simulink model "vehicle_model_controller_ref"  (R2020b)
settings: Solver=VariableStepAuto  StartTime=0.0  StopTime=180  FixedStep=0.001  RelTol=1e-3
model workspace (MAT data in the model file):
  understeer_gradient = 0.05
undefined symbols (not defined in the file or in its folder): front_forces, rear_forces
libraries: fl_lib x24, nesl_utility x20, sdl_lib x8, autolibmappedmotor x4, vehdynlibsteering x1, pid_lib x1, autolibshared x1, autolibdatasheetbattery x1
(part 1 of 4)
settings Model: TunableVars=F_sv,F_x_ij,F_x_ij_max,F_y_fl,F_y_fr,F_y_ij,F_y_rl,F_y_rr,J_z,K_1,K_2,LB,PID,R,T_x_ij,UP,delta,driver_input,err,l,l_f,l_r,linsol,s,s_f,s_r,x,x_1,x_2,x_3,x_4,y,y_1,y_2,y_3,y_4  TunableVarsStorageClass=Auto,Auto,Auto,Auto,Auto,Auto,Auto,Auto,Auto,Auto,Auto,Auto,Auto,Auto,Auto,Auto,Auto,Auto,Auto,Auto,Auto,Auto,Auto,Auto,Auto,Auto,Auto,Auto,Auto,Auto,Auto,Auto,Auto,Auto,Auto,Auto  TunableVarsTypeQualifier=,,,,,,,,,,,,,,,,,,,,,,,,,,,,,,,,,,,  ParameterArgumentNames=understeer_gradient  OrderedModelArguments=off  Creator=True  LastModifiedBy=Inver
settings DataIOCC: ExternalInput=Sheet1.getElement('driver_input'),Sheet1.getElement('batt_temp'),Sheet1.getElement('steering_angle'),Sheet1.getElement('wind z'),Sheet1.getElement('b_FL'),Sheet1.getElement('wind x'),Sheet1.getElement('wind y'),Sheet1.getElement('b_FR'),Sheet1.getElement('b_RL'),Sheet1.getElement('b_RR')  LoadExternalInput=on
settings OptimizationCC: DefaultParameterBehavior=Inlined  GainParamInheritBuiltInType=on  UseFloatMulNetSlope=on  InlineInvariantSignals=on  OptimizeBlockIOStorage=off  BufferReuse=off  EnhancedBackFolding=on  PassReuseOutputArgsThreshold=0  EfficientFloat2IntCast=on  EfficientMapNaN2IntZero=off  OptimizeBlockOrder=speed  DifferentSizesBufferReuse=on
settings DebuggingCC: SolverPrmCheckMsg=error  ParameterTunabilityLossMsg=error  ArithmeticOperatorsInVariantConditions=warning
settings HardwareCC: TargetBitPerPointer=64  TargetBitPerSizeT=64  TargetBitPerPtrDiffT=64  TargetLongLongMode=on  TargetIntDivRoundTo=Zero  TargetEndianess=LittleEndian  TargetWordSize=64  TargetHWDeviceType=MATLAB Host  ProdEqTarget=off
settings SFSimCC: SimUserIncludeDirs=$matlabroot$\toolbox\rtw\rtwdemos\EmbeddedCoderOverview\  SimAnalyzeCustomCode=on  MATLABDynamicMemAlloc=off  CustomCodeUndefinedFunction=UseInterfaceOnly  SimTargetLang=C++
settings RTWCC: Description=Rapid Simulation Target  SystemTargetFile=rsim.tlc  GenCodeOnly=on  TemplateMakefile=rsim_default_tmf  GenerateReport=on  BuildConfiguration=Faster Runs  LaunchReport=on  CheckMdlBeforeBuild=Warning
settings CodeAppCC: ForceParamTrailComments=on  OperatorAnnotations=on
settings RSimTargetCC: TargetLangStandard=C99 (ISO)
settings ConfigComp: CovScope=ReferencedModels
settings SimscapeCC: SimscapeLogType=local

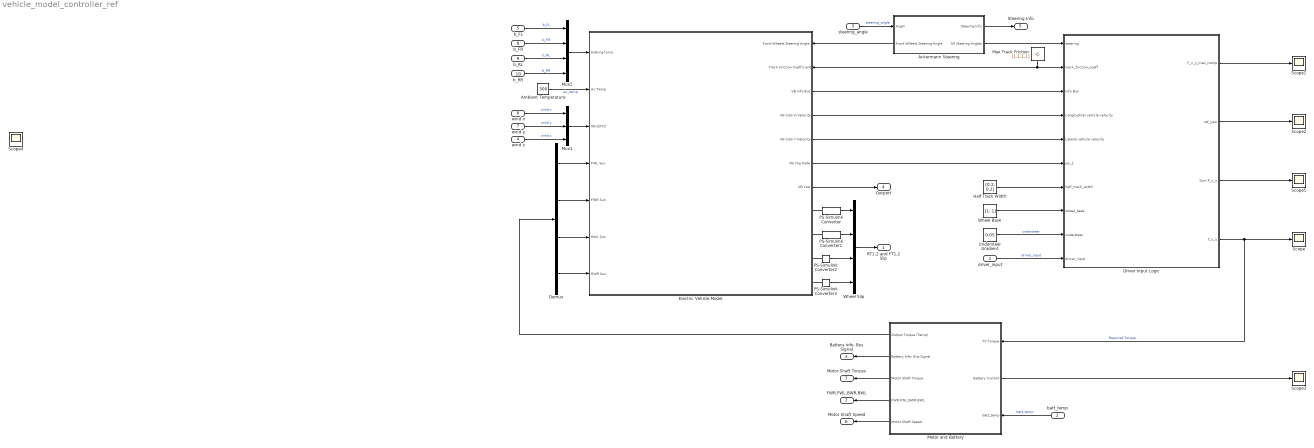
== system vehicle_model_controller_ref ==
  driver_input : Inport  Interpolate=off
  batt_temp : Inport  Port=2
  steering_angle : Inport  Port=3
  wind z : Inport  Port=4
  b_FL : Inport  Port=5
  wind x : Inport  Port=6
  wind y : Inport  Port=7
  b_FR : Inport  Port=8
  b_RL : Inport  Port=9
  b_RR : Inport  Port=10
  Ackermann Steering : Subsystem
      settings: PortSchema="{\"entries\":[{\"content\":{\"sides\":[{\"content\":{\"connectorIds\":[\"In1\",\"Out3\"]},\"type\":\"ConnectorPlacement.EquallySpacedRectSide\",\"uuid\":\"7629c306-c8a5-46d9-919e-1a99248f4fd8\"},{\"content\":{\"connectorIds\":[\"Out1\",\"Out2\"],\"side\":\"RIGHT\"},\"type\":\"ConnectorPlacement.EquallySpacedRectSide\",\"uuid\":\"a1deaca9-77cb-4ffb-842f-c827aa96d417\"},{\"content\":{\"connectorIds\":[],\"side\":\"TOP\"},\"type\":\"ConnectorPlacement.EquallySpacedRectSide\",\"uuid\":\"391c149d-58be-48e2-876e-8c407e7d25f9\"},{\"content\":{\"connectorIds\":[],\"side\":\"HIDDEN\"},\"type\":\"ConnectorPlacement.EquallySpacedRectSide\",\"uuid\":\"557ca4cc-9d5d-4724-8dd0-cdc929429066\"}]},\"type\":\"ConnectorPlacement.EquallySpacedConnector\",\"uuid\":\"b8a1e7c7-7192-4f65-ab36-8db1985dd1bc\"}],\"packageUris\":[\"http://schema.mathworks.com/mf0/Connector/R2020b\"],\"version\":\"1.0\"}"
  Ambient Temperature : Constant  Value=300
  Demux : Demux
  Driver Input Logic : Subsystem
  Electric Vehicle Model : Subsystem
      settings: PortSchema="{\"entries\":[{\"content\":{\"sides\":[{\"content\":{\"connectorIds\":[\"In1\",\"In2\",\"In3\",\"In4\",\"In5\",\"In6\",\"In7\"]},\"type\":\"ConnectorPlacement.EquallySpacedRectSide\",\"uuid\":\"d116468d-7868-487f-a964-21d40fbcc809\"},{\"content\":{\"connectorIds\":[\"In8\",\"In9\",\"Out1\",\"Out2\",\"Out3\",\"Out4\",\"Out5\",\"RConn1\",\"RConn2\",\"RConn3\",\"RConn4\"],\"side\":\"RIGHT\"},\"type\":\"ConnectorPlacement.EquallySpacedRectSide\",\"uuid\":\"69901164-3ba1-4787-94a1-b6dad3f5570f\"},{\"content\":{\"connectorIds\":[],\"side\":\"TOP\"},\"type\":\"ConnectorPlacement.EquallySpacedRectSide\",\"uuid\":\"0399aa14-7cbc-406a-a0bc-5234930aa618\"},{\"content\":{\"connectorIds\":[],\"side\":\"HIDDEN\"},\"type\":\"ConnectorPlacement.EquallySpacedRectSide\",\"uuid\":\"c7425876-ea80-44ac-a5c9-676a45313985\"}]},\"type\":\"ConnectorPlacement.EquallySpacedConnector\",\"uuid\":\"33585625-d9f5-41d4-8b4d-b29cb62e09b6\"}],\"packageUris\":[\"http://schema.mathworks.com/mf0/Connector/R2020b\"],\"version\":\"1.0\"}"
  Half Track Width : Constant  Value=[0.2, 0.2]
  Max Track Friction : Constant  Value=[1,1;1,1]
  Motor and Battery : Subsystem
      settings: PortSchema="{\"entries\":[{\"content\":{\"sides\":[{\"content\":{\"connectorIds\":[\"Out2\",\"Out3\",\"Out4\",\"Out5\",\"Out6\"]},\"type\":\"ConnectorPlacement.EquallySpacedRectSide\",\"uuid\":\"d5eb6e01-74de-485f-b814-f74cf87d6300\"},{\"content\":{\"connectorIds\":[\"In1\",\"Out1\",\"In2\"],\"side\":\"RIGHT\"},\"type\":\"ConnectorPlacement.EquallySpacedRectSide\",\"uuid\":\"4e9b95b3-1238-4789-a4cc-20b236b4d536\"},{\"content\":{\"connectorIds\":[],\"side\":\"TOP\"},\"type\":\"ConnectorPlacement.EquallySpacedRectSide\",\"uuid\":\"97fc91bc-a36c-43db-88cf-61ba0348fc60\"},{\"content\":{\"connectorIds\":[],\"side\":\"HIDDEN\"},\"type\":\"ConnectorPlacement.EquallySpacedRectSide\",\"uuid\":\"c955884f-22bb-4f22-9982-ff8bef63f64d\"}]},\"type\":\"ConnectorPlacement.EquallySpacedConnector\",\"uuid\":\"927982b2-ec40-42a1-9f55-58bc607d6a22\"}],\"packageUris\":[\"http://schema.mathworks.com/mf0/Connector/R2020b\"],\"version\":\"1.0\"}"
  Mux1 : Mux  Inputs=3
  Mux2 : Mux
  PS-Simulink Converter{,1..3} (4 alike) : nesl_utility/PS-Simulink Converter  PhysicalDomain=network_engine_domain  SubClassName=ps_output  LeftPortType=input  RightPortType=output  PseudoPeriodic=off  Frequencies=[]  Unit=inherit  AffineConversion=off
  Scope{,1..5} (6 alike) : Scope
  Understeer Gradient : Constant  Value=0.05
  Wheel Base : Constant  Value=[1, 1]
  Wheel Slip : Mux
  RT1,2 and FT1,2 Slip : Outport
  FWR,FWL,BWR,BWL : Outport  Port=2
  Battery Info- Bus Signal : Outport  Port=3
  Outport : Outport  Port=4
  Steering Info : Outport  Port=5
  Motor Shaft Speed : Outport  Port=6
  Motor Shaft Torque : Outport  Port=7
  wires:
  PS-Simulink Converter/1 -> Wheel Slip/1
  PS-Simulink Converter1/1 -> Wheel Slip/2
  PS-Simulink Converter2/1 -> Wheel Slip/3
  PS-Simulink Converter3/1 -> Wheel Slip/4
  Wheel Slip/1 -> RT1,2 and FT1,2 Slip/1
  Electric Vehicle Model/5(VB Yaw) -> Outport/1
  Ambient Temperature/1 -> Electric Vehicle Model/2(Air Temp)  "air_temp"
  Electric Vehicle Model/1(VB Info Bus) -> Driver Input Logic/3(Info Bus)
  Electric Vehicle Model/2("VB CoG X-Velocity ") -> Driver Input Logic/4(Longitudinal vehicle velocity)
  Electric Vehicle Model/3(VB CoG Y-Velocity) -> Driver Input Logic/5(Lateral vehicle velocity)
  Electric Vehicle Model/4(VB Yaw Rate) -> Driver Input Logic/6(psi_1)
  Understeer Gradient/1 -> Driver Input Logic/9(understeer)  "understeer"
  driver_input/1 -> Driver Input Logic/10(driver_input)  "driver_input"
  Driver Input Logic/4(T_x_ij) -> Scope/1, Motor and Battery/1(TV Torque)  "Required Torque"
  Half Track Width/1 -> Driver Input Logic/7(half_track_width)
  Wheel Base/1 -> Driver Input Logic/8(wheel_base)
  Driver Input Logic/1(F_x_ij_max_noslip) -> Scope1/1
  Driver Input Logic/2(ref_yaw) -> Scope2/1
  wind x/1 -> Mux1/1  "wind x"
  wind y/1 -> Mux1/2  "wind y"
  wind z/1 -> Mux1/3  "wind z"
  Mux1/1 -> Electric Vehicle Model/3(WindXYZ)
  b_FR/1 -> Mux2/2  "b_FR"
  b_FL/1 -> Mux2/1  "b_FL"
  b_RL/1 -> Mux2/3  "b_RL"
  b_RR/1 -> Mux2/4  "b_RR"
  Ackermann Steering/1(Steering Info) -> Steering Info/1
  Ackermann Steering/3(Front Wheels Steering Angle) -> Electric Vehicle Model/8(Front Wheels Steering Angle)
  Ackermann Steering/2(All Steering Angles) -> Driver Input Logic/1(steering)
  Max Track Friction/1 -> Driver Input Logic/2(track_friction_coeff), Electric Vehicle Model/9(Track Friction Coefficient)
  steering_angle/1 -> Ackermann Steering/1(AngIn)  "steering_angle"
  Driver Input Logic/3(Sum F_x_ij) -> Scope5/1
  Demux/4 -> Electric Vehicle Model/7(RWR Sun)
  Demux/3 -> Electric Vehicle Model/6(RWL Sun)
  Demux/2 -> Electric Vehicle Model/5(FWR Sun)
  Demux/1 -> Electric Vehicle Model/4(FWL Sun)
  Mux2/1 -> Electric Vehicle Model/1(braking force)
  batt_temp/1 -> Motor and Battery/2(batt_temp)  "batt_temp"
  Motor and Battery/2(Output Torque (Temp)) -> Demux/1
  Motor and Battery/1(Battery Current) -> Scope3/1
  Motor and Battery/3(Battery Info- Bus Signal) -> Battery Info- Bus Signal/1
  Motor and Battery/5(FWR,FWL,BWR,BWL) -> FWR,FWL,BWR,BWL/1
  Motor and Battery/4(Motor Shaft Torque) -> Motor Shaft Torque/1
  Motor and Battery/6(Motor Shaft Speed) -> Motor Shaft Speed/1
  connections:
  PS-Simulink Converter/LConn1 -- Electric Vehicle Model/RConn1
  PS-Simulink Converter1/LConn1 -- Electric Vehicle Model/RConn2
  PS-Simulink Converter2/LConn1 -- Electric Vehicle Model/RConn3
  PS-Simulink Converter3/LConn1 -- Electric Vehicle Model/RConn4

== system vehicle_model_controller_ref/Ackermann Steering ==
  AngIn : Inport
  Bus Creator : BusCreator  Inputs=2
  Deg to Rad : Gain  Gain=pi/180
  Kinematic Steering : vehdynlibsteering/Kinematic Steering  StrgType=Ackerman  StrgRatioType=Constant  Loc=Front  NrmlFctr=1  TrckWdth=1  WhlBase=1.524  Db=0  StrgRng=1.25*pi  StrgAngBpts="[-6.2832   -5.0265   -3.7699   -2.5133   -1.2566         0    1.2566    2.5133    3.7699    5.0265    6.2832]"  StrgRatioTbl=|  StrgRatio=1  StrgArmLngth=0.1  RckCsLngth=0.5  TieRodLngth=0.248  D=0.2  PnnRadius=0.0057  PnnRadiusTbl="[0.0055    0.0055    0.0056    0.0057    0.0058    0.0057    0.0057    0.0057    0.0056    0.0055    0.0055]"  RodLngth=0.1  ParaArmLngth=0.9  aMode=2
      | [13.5000   13.3750   13.2500   13.1250   13.0000   13.0000   13.0000   13.1250   13.2500   13.3750   13.5000
      | ]
  Mux3 : Mux  Inputs=2
  Steering Info : Outport
  All Steering Angles : Outport  Port=2
  Front Wheels Steering Angle : Outport  Port=3
  wires:
  Kinematic Steering/2 -> Mux3/1
  Kinematic Steering/3 -> Mux3/2
  Kinematic Steering/1 -> Steering Info/1
  Mux3/1 -> Bus Creator/1, Front Wheels Steering Angle/1  "ackermann angles"
  Bus Creator/1 -> All Steering Angles/1
  Deg to Rad/1 -> Kinematic Steering/1, Bus Creator/2  "steering_angle"
  AngIn/1 -> Deg to Rad/1  "steering_angle"

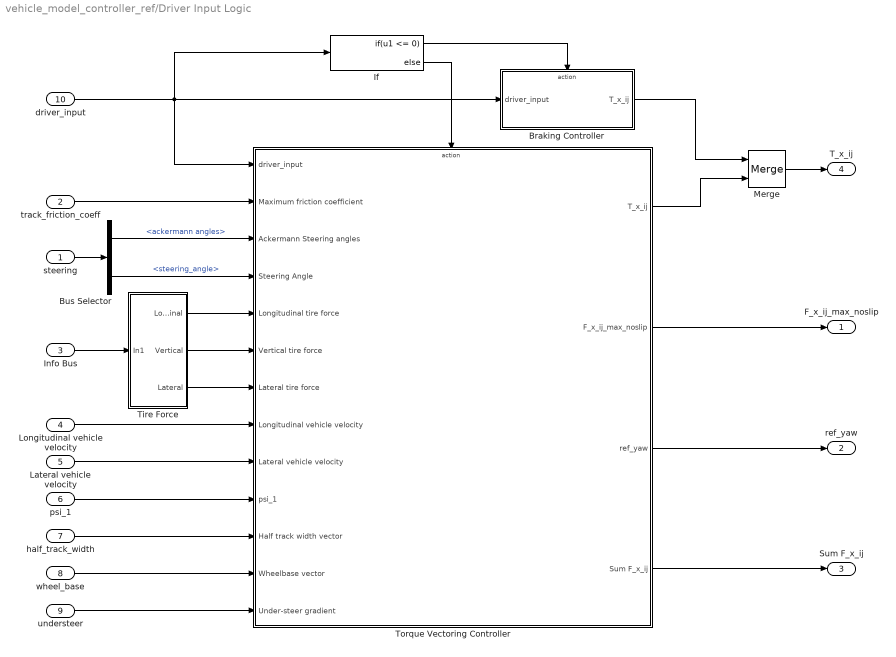
== system vehicle_model_controller_ref/Driver Input Logic ==
  steering : Inport
  track_friction_coeff : Inport  Port=2
  Info Bus : Inport  Port=3
  Longitudinal vehicle velocity : Inport  Port=4
  Lateral vehicle velocity : Inport  Port=5
  psi_1 : Inport  Port=6
  half_track_width : Inport  Port=7
  wheel_base : Inport  Port=8
  understeer : Inport  Port=9
  driver_input : Inport  Port=10
  Braking Controller : Subsystem
  Bus Selector : BusSelector  OutputSignals=ackermann angles,steering_angle
  If : If  IfExpression=u1 <= 0
  Merge : Merge
  Tire Force : Subsystem
  Torque Vectoring Controller : Subsystem
  F_x_ij_max_noslip : Outport
  ref_yaw : Outport  Port=2
  Sum F_x_ij : Outport  Port=3
  T_x_ij : Outport  Port=4
  wires:
  half_track_width/1 -> Torque Vectoring Controller/11(Half track width vector)
  understeer/1 -> Torque Vectoring Controller/13(Under-steer gradient)
  Tire Force/1(Longitudinal) -> Torque Vectoring Controller/5(Longitudinal tire force)
  Lateral vehicle velocity/1 -> Torque Vectoring Controller/9(Lateral vehicle velocity)
  wheel_base/1 -> Torque Vectoring Controller/12(Wheelbase vector)
  Longitudinal vehicle velocity/1 -> Torque Vectoring Controller/8(Longitudinal vehicle velocity)
  Tire Force/2(Vertical) -> Torque Vectoring Controller/6(Vertical tire force)
  Info Bus/1 -> Tire Force/1(In1)
  psi_1/1 -> Torque Vectoring Controller/10(psi_1)
  track_friction_coeff/1 -> Torque Vectoring Controller/2(Maximum friction coefficient)
  If/1 -> Braking Controller/Action
  Merge/1 -> T_x_ij/1
  If/2 -> Torque Vectoring Controller/Action
  Braking Controller/1(T_x_ij) -> Merge/1
  Torque Vectoring Controller/1(T_x_ij) -> Merge/2
  driver_input/1 -> Torque Vectoring Controller/1(driver_input), Braking Controller/1(driver_input), If/1
  Bus Selector/2 -> Torque Vectoring Controller/4(Steering Angle)  "<steering_angle>"
  Bus Selector/1 -> Torque Vectoring Controller/3("Ackermann Steering angles ")  "<ackermann angles>"
  Torque Vectoring Controller/2(F_x_ij_max_noslip) -> F_x_ij_max_noslip/1
  Torque Vectoring Controller/3(ref_yaw) -> ref_yaw/1
  Tire Force/3(Lateral) -> Torque Vectoring Controller/7(Lateral tire force)
  steering/1 -> Bus Selector/1
  Torque Vectoring Controller/4(Sum F_x_ij) -> Sum F_x_ij/1

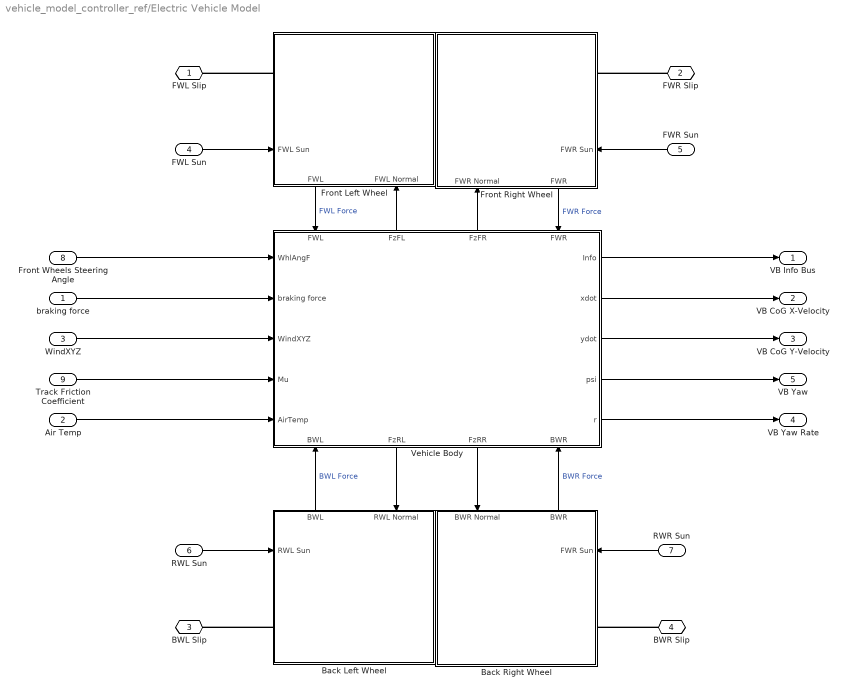
== system vehicle_model_controller_ref/Electric Vehicle Model ==
  braking force : Inport
  Air Temp : Inport  Port=2
  WindXYZ : Inport  Port=3
  FWL Sun : Inport  Port=4
  FWR Sun : Inport  Port=5
  RWL Sun : Inport  Port=6
  RWR Sun : Inport  Port=7
  Front Wheels Steering Angle : Inport  Port=8
  Track Friction Coefficient : Inport  Port=9
  Back Left Wheel : Subsystem
      settings: PortSchema="{\"entries\":[{\"content\":{\"sides\":[{\"content\":{\"connectorIds\":[\"In1\",\"LConn1\"]},\"type\":\"ConnectorPlacement.EquallySpacedRectSide\",\"uuid\":\"9f52900f-df3e-41ac-b258-782e5d4e0eaf\"},{\"content\":{\"connectorIds\":[],\"side\":\"RIGHT\"},\"type\":\"ConnectorPlacement.EquallySpacedRectSide\",\"uuid\":\"34c2d9dc-60c7-40ad-be28-599fbc039141\"},{\"content\":{\"connectorIds\":[\"Out1\",\"In2\"],\"side\":\"TOP\"},\"type\":\"ConnectorPlacement.EquallySpacedRectSide\",\"uuid\":\"1dcff801-acc8-4468-b9f1-4bf879f78c2b\"},{\"content\":{\"connectorIds\":[],\"side\":\"HIDDEN\"},\"type\":\"ConnectorPlacement.EquallySpacedRectSide\",\"uuid\":\"30765525-e7e6-43f5-8314-8ed292f1691c\"}]},\"type\":\"ConnectorPlacement.EquallySpacedConnector\",\"uuid\":\"fe63b2f8-6027-4789-9c90-5c54dbfc2a0a\"}],\"packageUris\":[\"http://schema.mathworks.com/mf0/Connector/R2020b\"],\"version\":\"1.0\"}"
  Back Right Wheel : Subsystem
      settings: PortSchema="{\"entries\":[{\"content\":{\"sides\":[{\"content\":{\"connectorIds\":[]},\"type\":\"ConnectorPlacement.EquallySpacedRectSide\",\"uuid\":\"9f52900f-df3e-41ac-b258-782e5d4e0eaf\"},{\"content\":{\"connectorIds\":[\"In2\",\"RConn1\"],\"side\":\"RIGHT\"},\"type\":\"ConnectorPlacement.EquallySpacedRectSide\",\"uuid\":\"34c2d9dc-60c7-40ad-be28-599fbc039141\"},{\"content\":{\"connectorIds\":[\"In1\",\"Out1\"],\"side\":\"TOP\"},\"type\":\"ConnectorPlacement.EquallySpacedRectSide\",\"uuid\":\"1dcff801-acc8-4468-b9f1-4bf879f78c2b\"},{\"content\":{\"connectorIds\":[],\"side\":\"HIDDEN\"},\"type\":\"ConnectorPlacement.EquallySpacedRectSide\",\"uuid\":\"30765525-e7e6-43f5-8314-8ed292f1691c\"}]},\"type\":\"ConnectorPlacement.EquallySpacedConnector\",\"uuid\":\"fe63b2f8-6027-4789-9c90-5c54dbfc2a0a\"}],\"packageUris\":[\"http://schema.mathworks.com/mf0/Connector/R2020b\"],\"version\":\"1.0\"}"
  Front Left Wheel : Subsystem
      settings: PortSchema="{\"entries\":[{\"content\":{\"sides\":[{\"content\":{\"connectorIds\":[\"LConn1\",\"In1\"]},\"type\":\"ConnectorPlacement.EquallySpacedRectSide\",\"uuid\":\"9f52900f-df3e-41ac-b258-782e5d4e0eaf\"},{\"content\":{\"connectorIds\":[],\"side\":\"RIGHT\"},\"type\":\"ConnectorPlacement.EquallySpacedRectSide\",\"uuid\":\"34c2d9dc-60c7-40ad-be28-599fbc039141\"},{\"content\":{\"connectorIds\":[],\"side\":\"TOP\"},\"type\":\"ConnectorPlacement.EquallySpacedRectSide\",\"uuid\":\"1dcff801-acc8-4468-b9f1-4bf879f78c2b\"},{\"content\":{\"connectorIds\":[\"Out1\",\"In2\"],\"side\":\"BOTTOM\"},\"type\":\"ConnectorPlacement.EquallySpacedRectSide\",\"uuid\":\"4fb396e2-b116-48bf-ae47-9a39d6e53df1\"},{\"content\":{\"connectorIds\":[],\"side\":\"HIDDEN\"},\"type\":\"ConnectorPlacement.EquallySpacedRectSide\",\"uuid\":\"30765525-e7e6-43f5-8314-8ed292f1691c\"}]},\"type\":\"ConnectorPlacement.EquallySpacedConnector\",\"uuid\":\"fe63b2f8-6027-4789-9c90-5c54dbfc2a0a\"}],\"packageUris\":[\"http://schema.mathworks.com/mf0/Connector/R2020b\"],\"version\":\"1.0\"}"
  Front Right Wheel : Subsystem
      settings: PortSchema="{\"entries\":[{\"content\":{\"sides\":[{\"content\":{\"connectorIds\":[]},\"type\":\"ConnectorPlacement.EquallySpacedRectSide\",\"uuid\":\"9f52900f-df3e-41ac-b258-782e5d4e0eaf\"},{\"content\":{\"connectorIds\":[\"RConn1\",\"In2\"],\"side\":\"RIGHT\"},\"type\":\"ConnectorPlacement.EquallySpacedRectSide\",\"uuid\":\"34c2d9dc-60c7-40ad-be28-599fbc039141\"},{\"content\":{\"connectorIds\":[],\"side\":\"TOP\"},\"type\":\"ConnectorPlacement.EquallySpacedRectSide\",\"uuid\":\"1dcff801-acc8-4468-b9f1-4bf879f78c2b\"},{\"content\":{\"connectorIds\":[\"In1\",\"Out1\"],\"side\":\"BOTTOM\"},\"type\":\"ConnectorPlacement.EquallySpacedRectSide\",\"uuid\":\"ca39b8f4-a765-4ff2-9936-a2d929862da7\"},{\"content\":{\"connectorIds\":[],\"side\":\"HIDDEN\"},\"type\":\"ConnectorPlacement.EquallySpacedRectSide\",\"uuid\":\"30765525-e7e6-43f5-8314-8ed292f1691c\"}]},\"type\":\"ConnectorPlacement.EquallySpacedConnector\",\"uuid\":\"fe63b2f8-6027-4789-9c90-5c54dbfc2a0a\"}],\"packageUris\":[\"http://schema.mathworks.com/mf0/Connector/R2020b\"],\"version\":\"1.0\"}"
  Vehicle Body : Subsystem
      settings: PortSchema="{\"entries\":[{\"content\":{\"sides\":[{\"content\":{\"connectorIds\":[\"In1\",\"In2\",\"In3\",\"In4\",\"In5\"]},\"type\":\"ConnectorPlacement.EquallySpacedRectSide\",\"uuid\":\"92155111-f8f4-4af5-b459-626db8603d20\"},{\"content\":{\"connectorIds\":[\"Out1\",\"Out2\",\"Out3\",\"Out4\",\"Out5\"],\"side\":\"RIGHT\"},\"type\":\"ConnectorPlacement.EquallySpacedRectSide\",\"uuid\":\"ae116824-7c15-47a3-8409-e548e47da19f\"},{\"content\":{\"connectorIds\":[\"In6\",\"Out8\",\"Out9\",\"In7\"],\"side\":\"TOP\"},\"type\":\"ConnectorPlacement.EquallySpacedRectSide\",\"uuid\":\"47f131ff-f47a-4e72-9486-74af6f2f1ac7\"},{\"content\":{\"connectorIds\":[\"In8\",\"Out6\",\"Out7\",\"In9\"],\"side\":\"BOTTOM\"},\"type\":\"ConnectorPlacement.EquallySpacedRectSide\",\"uuid\":\"2f2033fb-4ff2-47eb-b510-cc1663364d24\"},{\"content\":{\"connectorIds\":[],\"side\":\"HIDDEN\"},\"type\":\"ConnectorPlacement.EquallySpacedRectSide\",\"uuid\":\"f9b1c4a7-012e-4646-ac9d-ce6bcd7dfdc6\"}]},\"type\":\"ConnectorPlacement.EquallySpacedConnector\",\"uuid\":\"6b8ecd22-cccf-4b6d-aa41-24252124a118\"}],\"packageUris\":[\"http://schema.mathworks.com/mf0/Connector/R2020b\"],\"version\":\"1.0\"}"
  FWL Slip : PMIOPort  Side=Right
  FWR Slip : PMIOPort  Port=2  Side=Right
  BWL Slip : PMIOPort  Port=3  Side=Right
  BWR Slip : PMIOPort  Port=4  Side=Right
  VB Info Bus : Outport
  "VB CoG X-Velocity " : Outport  Port=2
  VB CoG Y-Velocity : Outport  Port=3
  VB Yaw Rate : Outport  Port=4
  VB Yaw : Outport  Port=5  OutDataTypeStr=double
  wires:
  Front Wheels Steering Angle/1 -> Vehicle Body/1(WhlAngF)
  WindXYZ/1 -> Vehicle Body/3(WindXYZ)
  Track Friction Coefficient/1 -> Vehicle Body/4(Mu)
  Air Temp/1 -> Vehicle Body/5(AirTemp)
  Vehicle Body/1(Info) -> VB Info Bus/1
  Vehicle Body/2(xdot) -> "VB CoG X-Velocity "/1
  Vehicle Body/3(ydot) -> VB CoG Y-Velocity/1
  Front Left Wheel/1(FWL) -> Vehicle Body/6(FWL)  "FWL Force"
  braking force/1 -> Vehicle Body/2(braking force)
  Back Left Wheel/1(BWL) -> Vehicle Body/8(BWL)  "BWL Force"
  Back Right Wheel/1(BWR) -> Vehicle Body/9(BWR)  "BWR Force"
  Front Right Wheel/1(FWR) -> Vehicle Body/7(FWR)  "FWR Force"
  Vehicle Body/9(FzFR) -> Front Right Wheel/1(FWR Normal)
  Vehicle Body/8(FzFL) -> Front Left Wheel/2(FWL Normal)
  Vehicle Body/6(FzRL) -> Back Left Wheel/2(RWL Normal)
  Vehicle Body/7(FzRR) -> Back Right Wheel/1(BWR Normal)
  Vehicle Body/4(psi) -> VB Yaw/1
  Vehicle Body/5(r) -> VB Yaw Rate/1
  FWL Sun/1 -> Front Left Wheel/1(FWL Sun)
  FWR Sun/1 -> Front Right Wheel/2(FWR Sun)
  RWL Sun/1 -> Back Left Wheel/1(RWL Sun)
  RWR Sun/1 -> Back Right Wheel/2(FWR Sun)
  connections:
  Back Left Wheel/LConn1 -- BWL Slip/RConn1
  BWR Slip/RConn1 -- Back Right Wheel/RConn1
  Front Left Wheel/LConn1 -- FWL Slip/RConn1
  FWR Slip/RConn1 -- Front Right Wheel/RConn1

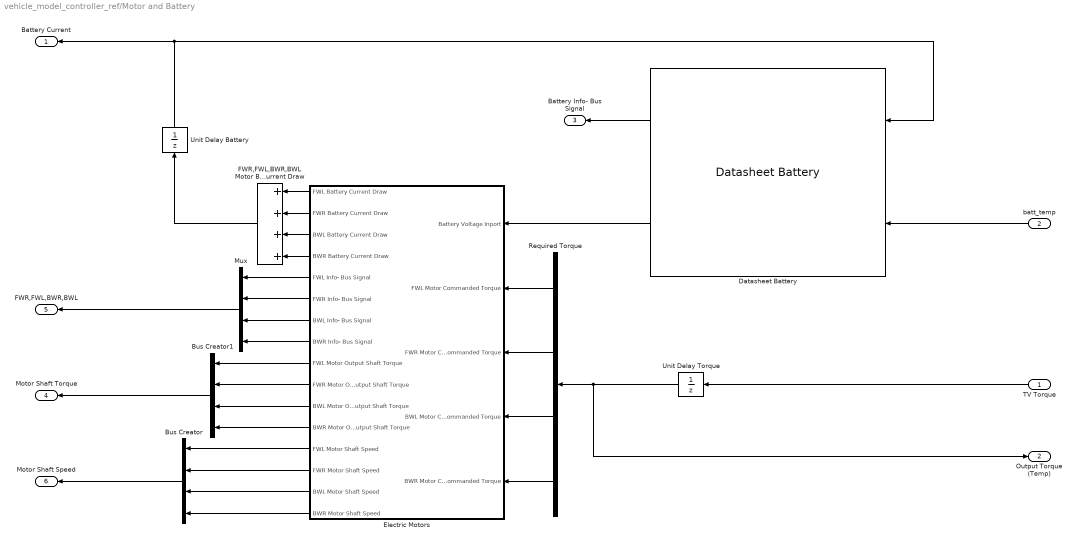
== system vehicle_model_controller_ref/Motor and Battery ==
  TV Torque : Inport
  batt_temp : Inport  Port=2
  Bus Creator : BusCreator  Inputs=FWL Speed,FWR Speed,BWL Speed,BWR Speed
  Bus Creator1 : BusCreator  Inputs=FWL Torque,FWR Torque,BWL Torque,BWR Torque
  Datasheet Battery : autolibdatasheetbattery/Datasheet Battery  CapacityCtrl=Parameter  OutputVlt=Unfiltered  BattChargeMax=32.5  Em=[2.8 3.228 3.284 3.361 3.408 3.427 3.472 3.477 3.493 3.504 3.516 3.528 3.537 3.545 3.555 3.561 3.566 3.576 3.587 3.589 3.594 3.6 3.608 3.61 3.616 3.619 3.626 3.632 3.637 3.64 3.645 3.646 3.652 3.655 3.658 3.661 3.664 3.668 3.673 3.678 3.68 3.681 3.686 3.692 3.699 3.702 3.705 3.71 3.717 3.723 3.728 3.733 3.735 3.742 3.749 3.755 3.761 3.768 3.773 3.78 3.791 3.798 3.798 3.814 3.818 3.825 3.841 3.846 3.855 3.863 3.877 3.885 3.894 3.907 3.919 3.926 3.935 3.944 3.954 3.964 3.974 3.988 3.998 4.014 4.029 4.034 4.047 4.065 4.074 4.086 4.097 4.131 4.126 4.138 4.15 4.18 4.174 4.187 4.207 4.231 4.221]  CapLUTBp=[0 0.01 0.02 0.03 0.04 0.05 0.06 0.07 0.08 0.09 0.1 0.11 0.12 0.13 0.14 0.15 0.16 0.17 0.18 0.19 0.2 0.21 0.22 0.23 0.24 0.25 0.26 0.27 0.28 0.29 0.3 0.31 0.32 0.33 0.34 0.35 0.36 0.37 0.38 0.39 0.4 0.41 0.42 0.43 0.44 0.45 0.46 0.47 0.48 0.49 0.5 0.51 0.52 0.53 0.54 0.55 0.56 0.57 0.58 0.59 0.6 0.61 0.62 0.63 0.64 0.65 0.66 0.67 0.68 0.69 0.7 0.71 0.72 0.73 0.74 0.75 0.76 0.77 0.78 0.79 0.8 0.81 0.82 0.83 0.84 0.85 0.86 0.87 0.88 0.89 0.9 0.91 0.92 0.93 0.94 0.95 0.96 0.97 0.98 0.99 1]  RInt=[0.008846 0.009319 0.009027 0.00847 0.01032 0.01314;0.006389 0.006554 0.005553 0.005525 0.006043 0.007805;0.004364 0.004101 0.00406 0.003452 0.003846 0.004517;0.002031 0.002563 0.002532 0.00246 0.002716 0.003047;0.001443 0.001825 0.001795 0.001778 0.001924 0.002234;0.0005603 0.0007192 0.0006887 0.0007557 0.0007355 0.001014;0.001028 0.001338 0.001 0.001536 0.001546 0.002789]  BattTempBp=[243.1 253.1 263.1 273.1 283.1 298.1 313.1]  CapSOCBp=[0 0.2 0.4 0.6 0.8 1]  Ns=96  Np=2  BattCapInit=26  Tc=1/1000  Vinit=4.221  RefBlkName='autolibdatasheetbattery/Datasheet Battery'
      settings: SourceProductBaseCode=PW
  Electric Motors : Subsystem
  FWR,FWL,BWR,BWL Motor Battery Current Draw : Sum  Inputs=++++
  Mux : Mux
  Required Torque : Demux
  Unit Delay Battery : UnitDelay  SampleTime=-1  HasFrameUpgradeWarning=on
  Unit Delay Torque : UnitDelay  SampleTime=-1  HasFrameUpgradeWarning=on
  Battery Current : Outport
  Output Torque (Temp) : Outport  Port=2
  Battery Info- Bus Signal : Outport  Port=3
  Motor Shaft Torque : Outport  Port=4
  FWR,FWL,BWR,BWL : Outport  Port=5
  Motor Shaft Speed : Outport  Port=6
  wires:
  Bus Creator1/1 -> Motor Shaft Torque/1
  Mux/1 -> FWR,FWL,BWR,BWL/1
  Required Torque/3 -> Electric Motors/4(BWL Motor Commanded Torque)
  Electric Motors/3(BWL Battery Current Draw) -> FWR,FWL,BWR,BWL Motor Battery Current Draw/3
  Required Torque/2 -> Electric Motors/3("FWR Motor Commanded Torque ")
  Required Torque/1 -> Electric Motors/2(FWL Motor Commanded Torque)
  Datasheet Battery/2 -> Electric Motors/1(Battery Voltage Inport)
  Datasheet Battery/1 -> Battery Info- Bus Signal/1
  Electric Motors/12(BWR Motor Output Shaft Torque) -> Bus Creator1/4
  Required Torque/4 -> Electric Motors/5(BWR Motor Commanded Torque)
  Unit Delay Battery/1 -> Datasheet Battery/1, Battery Current/1
  Bus Creator/1 -> Motor Shaft Speed/1
  Electric Motors/5(FWL Info- Bus Signal) -> Mux/1
  batt_temp/1 -> Datasheet Battery/2
  Electric Motors/1(FWL Battery Current Draw) -> FWR,FWL,BWR,BWL Motor Battery Current Draw/1
  FWR,FWL,BWR,BWL Motor Battery Current Draw/1 -> Unit Delay Battery/1
  Electric Motors/15(BWL Motor Shaft Speed) -> Bus Creator/3
  Electric Motors/6(FWR Info- Bus Signal) -> Mux/2
  Electric Motors/16(BWR Motor Shaft Speed) -> Bus Creator/4
  Unit Delay Torque/1 -> Output Torque (Temp)/1, Required Torque/1
  Electric Motors/14(FWR Motor Shaft Speed) -> Bus Creator/2
  Electric Motors/2(FWR Battery Current Draw) -> FWR,FWL,BWR,BWL Motor Battery Current Draw/2
  Electric Motors/11(BWL Motor Output Shaft Torque) -> Bus Creator1/3
  Electric Motors/13(FWL Motor Shaft Speed) -> Bus Creator/1
  Electric Motors/7(BWL Info- Bus Signal) -> Mux/3
  Electric Motors/9(FWL Motor Output Shaft Torque) -> Bus Creator1/1
  Electric Motors/8(BWR Info- Bus Signal) -> Mux/4
  Electric Motors/4(BWR Battery Current Draw) -> FWR,FWL,BWR,BWL Motor Battery Current Draw/4
  Electric Motors/10(FWR Motor Output Shaft Torque) -> Bus Creator1/2
  TV Torque/1 -> Unit Delay Torque/1

== system vehicle_model_controller_ref/Driver Input Logic/Braking Controller ==
  driver_input : Inport
  Action Port : ActionPort  InitializeStates=reset  PropagateVarSize=During execution  ActionPortLabel=if(u1 <= 0)
  MATLAB Function : MATLAB Function  TreatAsAtomicUnit=on
  T_x_ij : Outport
  wires:
  driver_input/1 -> MATLAB Function/1(driver_input)
  MATLAB Function/1(T_x_ij) -> T_x_ij/1

== system vehicle_model_controller_ref/Driver Input Logic/Tire Force ==
  In1 : Inport
  Bus Selector : BusSelector  OutputSignals=BdyFrm.Forces.RearAxl.Rght.Fx,BdyFrm.Forces.RearAxl.Lft.Fx,BdyFrm.Forces.FrntAxl.Rght.Fx,BdyFrm.Forces.FrntAxl.Lft.Fx,BdyFrm.Forces.RearAxl.Rght.Fz,BdyFrm.Forces.RearAxl.Lft.Fz,BdyFrm.Forces.FrntAxl.Rght.Fz,BdyFrm.Forces.FrntAxl.Lft.Fz,BdyFrm.Forces.FrntAxl.Lft.Fy,BdyFrm.Forces.FrntAxl.Rght.Fy,BdyFrm.Forces.RearAxl.Lft.Fy,BdyFrm.Forces.RearAxl.Rght.Fy
  Mux1 : Mux
  Mux6 : Mux
  Mux7 : Mux
  Longitudinal : Outport
  Vertical : Outport  Port=2
  Lateral : Outport  Port=3
  wires:
  Bus Selector/2 -> Mux6/2  "<Fx>"
  Bus Selector/8 -> Mux7/4  "<Fz>"
  Bus Selector/5 -> Mux7/1  "<Fz>"
  Bus Selector/6 -> Mux7/2  "<Fz>"
  Bus Selector/1 -> Mux6/1  "<Fx>"
  Mux6/1 -> Longitudinal/1
  Bus Selector/4 -> Mux6/4  "<Fx>"
  Bus Selector/3 -> Mux6/3  "<Fx>"
  Bus Selector/7 -> Mux7/3  "<Fz>"
  Mux7/1 -> Vertical/1
  In1/1 -> Bus Selector/1
  Mux1/1 -> Lateral/1
  Bus Selector/9 -> Mux1/1  "<Fy>"
  Bus Selector/10 -> Mux1/2  "<Fy>"
  Bus Selector/11 -> Mux1/3  "<Fy>"
  Bus Selector/12 -> Mux1/4  "<Fy>"

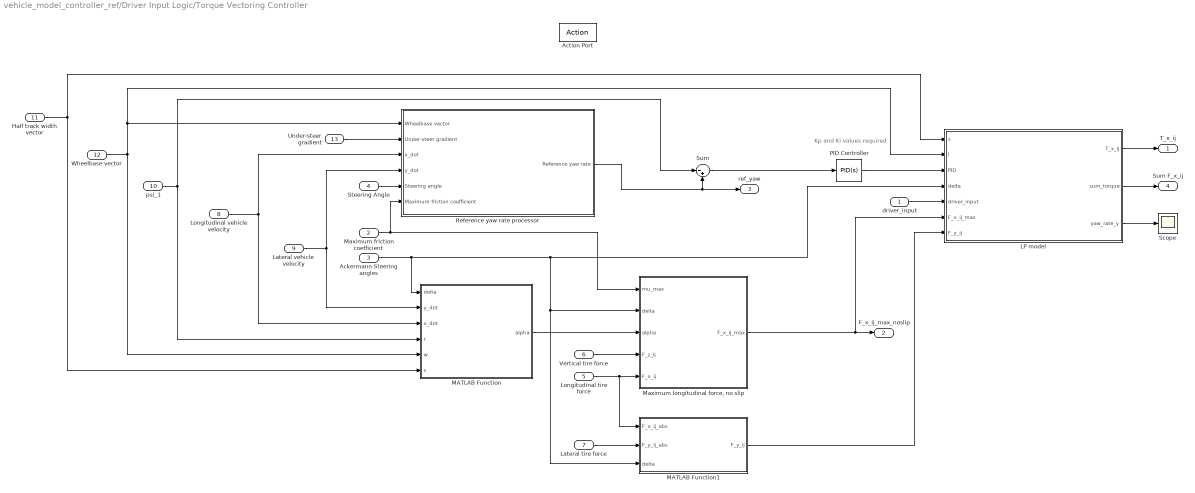
== system vehicle_model_controller_ref/Driver Input Logic/Torque Vectoring Controller ==
  note: Kp and Ki values required
  driver_input : Inport
  Maximum friction coefficient : Inport  Port=2
  "Ackermann Steering angles " : Inport  Port=3
  Steering Angle : Inport  Port=4
  Longitudinal tire force : Inport  Port=5
  Vertical tire force : Inport  Port=6
  Lateral tire force : Inport  Port=7
  Longitudinal vehicle velocity : Inport  Port=8
  Lateral vehicle velocity : Inport  Port=9
  psi_1 : Inport  Port=10
  Half track width vector : Inport  Port=11
  Wheelbase vector : Inport  Port=12
  Under-steer gradient : Inport  Port=13
  Action Port : ActionPort  InitializeStates=reset  PropagateVarSize=During execution  ActionPortLabel=else
  LP model : MATLAB Function  TreatAsAtomicUnit=on
  MATLAB Function : MATLAB Function  TreatAsAtomicUnit=on
  MATLAB Function1 : MATLAB Function  TreatAsAtomicUnit=on
  "Maximum longitudinal force, no slip" : MATLAB Function  TreatAsAtomicUnit=on
  PID Controller : pid_lib/PID Controller  Controller=PID  Form=Parallel  TimeDomain=Continuous-time  UseExternalTs=off  SampleTime=-1  IntegratorMethod=Forward Euler  FilterMethod=Forward Euler  ControllerParametersSource=internal  P=20  I=3  D=0  UseFilter=on  N=100  TunerSelectOption=Transfer Function Based (PID Tuner App)  InitialConditionSource=internal  InitialConditionForIntegrator=0  InitialConditionForFilter=0  DifferentiatorICPrevScaledInput=0  ExternalReset=none  TrackingMode=off  Kt=1  LimitOutput=on  SatLimitsSource=internal  UpperSaturationLimit=inf  LowerSaturationLimit=-inf  LinearizeAsGain=on  AntiWindupMode=none  Kb=1  POutMin=[]  POutMax=[]  IOutMin=[]  IOutMax=[]  DOutMin=[]  DOutMax=[]  NOutMin=[]  NOutMax=[]  SumOutMin=[]  SumOutMax=[]  SaturationOutMin=[]  SaturationOutMax=[]  PParamMin=[]  PParamMax=[]  IParamMin=[]  IParamMax=[]  DParamMin=[]  DParamMax=[]  NParamMin=[]  NParamMax=[]  KbParamMin=[]  KbParamMax=[]  KtParamMin=[]  KtParamMax=[]  KbOutMin=[]  KbOutMax=[]  KtOutMin=[]  KtOutMax=[]  IntegratorOutMin=[]  IntegratorOutMax=[]  FilterOutMin=[]  FilterOutMax=[]  SumI1OutMin=[]  SumI1OutMax=[]  SumI2OutMin=[]  SumI2OutMax=[]  SumI3OutMin=[]  SumI3OutMax=[]  SumI4OutMin=[]  SumI4OutMax=[]  SumDOutMin=[]  SumDOutMax=[]  DifferentiatorOutMin=[]  DifferentiatorOutMax=[]  FilterDiffOutCoefMin=[]  FilterDiffOutCoefMax=[]  ReciprocalOutMin=[]  ReciprocalOutMax=[]  SumDenOutMin=[]  SumDenOutMax=[]  SumNumOutMin=[]  SumNumOutMax=[]  DivideOutMin=[]  DivideOutMax=[]  UdiffTsProdOutMin=[]  UdiffTsProdOutMax=[]  NTsProdOutMin=[]  NTsProdOutMax=[]  UintegralTsProdOutMin=[]  UintegralTsProdOutMax=[]  UngainTsProdOutMin=[]  UngainTsProdOutMax=[]  IntegratorContinuousStateAttributes=''  IntegratorStateMustResolveToSignalObject=off  IntegratorRTWStateStorageClass=Auto  FilterContinuousStateAttributes=''  FilterStateMustResolveToSignalObject=off  FilterRTWStateStorageClass=Auto  ParallelPVariant=InternalParameters  IdealPVariant=Disabled  IVariant=InternalParameters  DVariant=InternalParameters  IntegratorVariant=Continuous  SatVariant=Enabled  AWVariant=Passthrough  PCopyVariant=Disabled  TRVariant=Disabled  FdbkBlocksVariant=Forward  IdealPFdbkVariant=Disabled  SatFdbkVariant=Disabled  DerivativeFilterVariant=ContFilter  NVariant=InternalParameters  NCopyVariant=Disabled  FilterICVariant=InternalICsFilter  IntegratorICVariant=InternalICs  ExternalResetVariant=Disabled  TRSumVariant=Passthrough  SumFdbkVariant=Disabled  SumVariant=Sum_PID  TsampFilterVariant=InternalTs  TsampNgainVariant=Passthrough  TsampIntegralVariant=Passthrough  ExternalSaturationOutDataTypeStr=Inherit: Same as second input
  Reference yaw rate processor : Subsystem
  Scope : Scope
  Sum : Sum  Inputs=|-+
  T_x_ij : Outport
  F_x_ij_max_noslip : Outport  Port=2
  ref_yaw : Outport  Port=3
  Sum F_x_ij : Outport  Port=4
  wires:
  PID Controller/1 -> LP model/3(PID)
  Maximum friction coefficient/1 -> Reference yaw rate processor/6(Maximum friction coefficient), "Maximum longitudinal force, no slip"/1(mu_max)
  Under-steer gradient/1 -> Reference yaw rate processor/2(Under-steer gradient)
  Reference yaw rate processor/1(Reference yaw rate) -> ref_yaw/1, Sum/2
  Sum/1 -> PID Controller/1
  Half track width vector/1 -> LP model/1(s), MATLAB Function/6(s)
  Wheelbase vector/1 -> Reference yaw rate processor/1(Wheelbase vector), LP model/2(l), MATLAB Function/5(w)
  "Maximum longitudinal force, no slip"/1(F_x_ij_max) -> F_x_ij_max_noslip/1, LP model/6(F_x_ij_max)
  Longitudinal tire force/1 -> "Maximum longitudinal force, no slip"/5(F_x_ij), MATLAB Function1/1(F_x_ij_abs)
  Vertical tire force/1 -> "Maximum longitudinal force, no slip"/4(F_z_ij)
  MATLAB Function/1(alpha) -> "Maximum longitudinal force, no slip"/3(alpha)
  Longitudinal vehicle velocity/1 -> Reference yaw rate processor/3(x_dot), MATLAB Function/3(x_dot)
  Lateral vehicle velocity/1 -> Reference yaw rate processor/4(y_dot), MATLAB Function/2(y_dot)
  "Ackermann Steering angles "/1 -> LP model/4(delta), "Maximum longitudinal force, no slip"/2(delta), MATLAB Function1/3(delta), MATLAB Function/1(delta)
  Steering Angle/1 -> Reference yaw rate processor/5("Steering angle ")
  MATLAB Function1/1(F_y_ij) -> LP model/7(F_y_ij)
  Lateral tire force/1 -> MATLAB Function1/2(F_y_ij_abs)
  driver_input/1 -> LP model/5(driver_input)
  LP model/1(T_x_ij) -> T_x_ij/1
  psi_1/1 -> MATLAB Function/4(r), Sum/1
  LP model/2(sum_torque) -> Sum F_x_ij/1
  LP model/3(yaw_rate_y) -> Scope/1

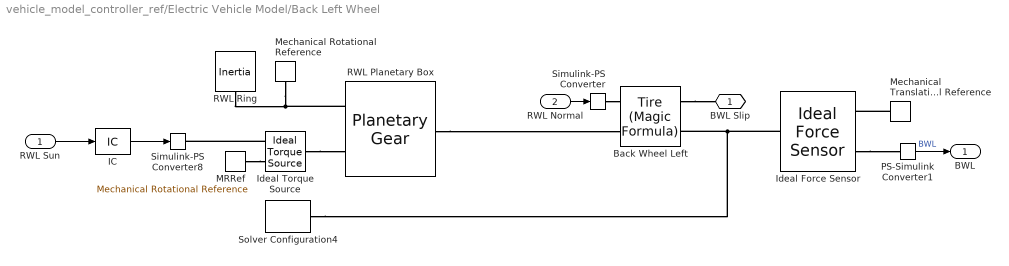
== system vehicle_model_controller_ref/Electric Vehicle Model/Back Left Wheel ==
  RWL Sun : Inport
  RWL Normal : Inport  Port=2
  Back Wheel Left : sdl_lib/Tires & Vehicles/Tire (Magic Formula)  parameterization=sdl.enum.magic_tire_model.peak  F_z1=3000 N  F_x1=3500 N  kappa1=10  B_m=10  C_m=1.9  D_m=1  E_m=0.97  fz0=4000 N  p_Cx=1.685  p_Dx=[1.21, -.037]  p_Ex=[.344, .095, -.02, 0]  p_Kx=[21.51, -.163, .245]  p_Hx=[-.002, .002]  p_Vx=[0, 0]  v_tr_thr=0.1 m/s  r_e=0.3 m  model_compliance=0  stiffness=1e6 N/m  damping=1000 N/(m/s)  model_inertia=0  inertia=1 kg*m^2  initial_velocity=0 rad/s  model_resistance=0  resistance_model=1  coeff=0.015  p_tire=250e3 Pa  alpha=-0.003  beta=0.97  coeff_a=84e-4  coeff_b=6.2e-4 s/m  coeff_c=1.6e-4 s^2/m^2  v_thr=0.001 m/s
  IC : InitialCondition  Value=0
  Ideal Force Sensor : fl_lib/Mechanical/Mechanical Sensors/Ideal Force Sensor
  Ideal Torque Source : fl_lib/Mechanical/Mechanical Sources/Ideal Torque Source
      settings: SourceProductName=Foundation Library
  MRRef : fl_lib/Mechanical/Rotational Elements/Mechanical Rotational Reference
      settings: SourceProductName=Foundation Library
  Mechanical Rotational Reference : fl_lib/Mechanical/Rotational Elements/Mechanical Rotational Reference
  Mechanical Translational Reference : fl_lib/Mechanical/Translational Elements/Mechanical Translational Reference
  PS-Simulink Converter1 : nesl_utility/PS-Simulink Converter  PhysicalDomain=network_engine_domain  SubClassName=ps_output  LeftPortType=input  RightPortType=output  PseudoPeriodic=off  Frequencies=[]  Unit=N  AffineConversion=off
  RWL Planetary Box : sdl_lib/Gears/Planetary Gear  rs_ratio=5.5  friction_model=sdl.enum.gear_friction.none  mu_visc=[0.01, 0.01] N*m/(rad/s)  efficiency=[.96, .98]  temperature_TLU=[280, 300, 320] K  efficiency_sp_TLU=[.95, .9, .85]  efficiency_rp_TLU=[.95, .9, .85]  pwr_thr=[.001, .001] W  thermal_mass=50 J/K  T_init=300 K  model_inertia=simscape.enum.onoff.off  planet_inertia=0.001 kg*m^2
      settings: SourceProductBaseCode=LD  LogSimulationData=on
  RWL Ring : fl_lib/Mechanical/Rotational Elements/Inertia  inertia=0.1 kg*m^2  num_ports=foundation.enum.numPorts2.one  w_specify=off  w_priority=High  w=0 rad/s  w_nominal_specify=off  w_nominal_unit=rad/s  w_nominal_value=1  t_specify=off  t_priority=None  t=0 N*m  t_nominal_specify=off  t_nominal_unit=N*m  t_nominal_value=1
  Simulink-PS Converter : nesl_utility/Simulink-PS Converter  PhysicalDomain=network_engine_domain  SubClassName=ps_input  LeftPortType=input  RightPortType=output  PseudoPeriodic=off  Frequencies=[]  NoiseDistribution=none  NoiseParameters=[]  Unit=N  AffineConversion=off  FilteringAndDerivatives=zero  SimscapeFilterOrder=1  InputFilterTimeConstant=0.001  UdotUserProvided=0
  Simulink-PS Converter8 : nesl_utility/Simulink-PS Converter  PhysicalDomain=network_engine_domain  SubClassName=ps_input  LeftPortType=input  RightPortType=output  PseudoPeriodic=off  Frequencies=[]  NoiseDistribution=none  NoiseParameters=[]  Unit=N*m  AffineConversion=off  FilteringAndDerivatives=zero  SimscapeFilterOrder=1  InputFilterTimeConstant=0.001  UdotUserProvided=0
  Solver Configuration4 : nesl_utility/Solver Configuration  PhysicalDomain=network_engine_domain  SubClassName=solver  LeftPortType=input  RightPortType=generic  Tones=[]  Harmonics=[]  SimulateNoise=off  Profile=off  UseLocalSampling=off  EnableSwitchedLinearOptims=on  FrequencyDomain=off  UseCCode=off  RelTol=0.001  AbsTol=1e-06  MinStep=1e-09  ToWorkspace=off  RevertToSquareIcSolve=off  NumHomotopyIterations=100  PhasorMode=off  PhasorModeNumHarmonics=1  DoDC=on  ResidualTolerance=1e-09  UseLocalSolver=off  LocalSolverChoice=NE_BACKWARD_EULER_ADVANCER  LocalSolverSampleTime=0.001  DoFixedCost=off  MaxNonlinIter=3  MaxModeIter=2  ComputeImpulses=off  ImpulseIterations=2  LinearAlgebra=auto  EquationFormulation=NE_TIME_EF  DelaysMemoryBudget=1024  AutomaticFiltering=on  FilteringTimeConstant=0.001  PartitionStorageMethod=AS_NEEDED  PartitionMemoryBudget=1024  PartitionMethod=ROBUST
  BWL Slip : PMIOPort  Side=Left
  BWL : Outport
  wires:
  PS-Simulink Converter1/1 -> BWL/1  "BWL"
  RWL Normal/1 -> Simulink-PS Converter/1
  IC/1 -> Simulink-PS Converter8/1
  RWL Sun/1 -> IC/1
  connections:
  Back Wheel Left/RConn1 -- BWL Slip/RConn1
  RWL Planetary Box/LConn1 -- Back Wheel Left/LConn2
  Ideal Force Sensor/RConn2 -- PS-Simulink Converter1/LConn1
  Ideal Force Sensor/LConn1 -- Solver Configuration4/RConn1 -- Back Wheel Left/RConn2
  Simulink-PS Converter/RConn1 -- Back Wheel Left/LConn1
  Mechanical Translational Reference/LConn1 -- Ideal Force Sensor/RConn1
  Mechanical Rotational Reference/LConn1 -- RWL Ring/LConn1 -- RWL Planetary Box/RConn1
  MRRef/LConn1 -- Ideal Torque Source/RConn2
  Ideal Torque Source/LConn1 -- RWL Planetary Box/RConn2
  Ideal Torque Source/RConn1 -- Simulink-PS Converter8/RConn1

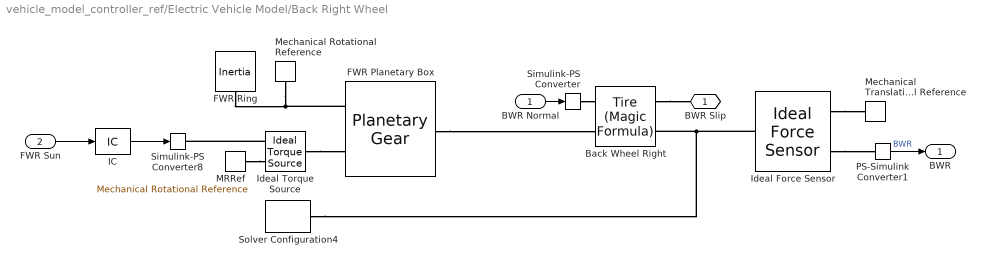
== system vehicle_model_controller_ref/Electric Vehicle Model/Back Right Wheel ==
  BWR Normal : Inport
  FWR Sun : Inport  Port=2
  Back Wheel Right : sdl_lib/Tires & Vehicles/Tire (Magic Formula)  parameterization=sdl.enum.magic_tire_model.peak  F_z1=3000 N  F_x1=3500 N  kappa1=10  B_m=10  C_m=1.9  D_m=1  E_m=0.97  fz0=4000 N  p_Cx=1.685  p_Dx=[1.21, -.037]  p_Ex=[.344, .095, -.02, 0]  p_Kx=[21.51, -.163, .245]  p_Hx=[-.002, .002]  p_Vx=[0, 0]  v_tr_thr=0.1 m/s  r_e=0.3 m  model_compliance=0  stiffness=1e6 N/m  damping=1000 N/(m/s)  model_inertia=0  inertia=1 kg*m^2  initial_velocity=0 rad/s  model_resistance=0  resistance_model=1  coeff=0.015  p_tire=250e3 Pa  alpha=-0.003  beta=0.97  coeff_a=84e-4  coeff_b=6.2e-4 s/m  coeff_c=1.6e-4 s^2/m^2  v_thr=0.001 m/s
  FWR Planetary Box : sdl_lib/Gears/Planetary Gear  rs_ratio=5.5  friction_model=sdl.enum.gear_friction.none  mu_visc=[0.01, 0.01] N*m/(rad/s)  efficiency=[.96, .98]  temperature_TLU=[280, 300, 320] K  efficiency_sp_TLU=[.95, .9, .85]  efficiency_rp_TLU=[.95, .9, .85]  pwr_thr=[.001, .001] W  thermal_mass=50 J/K  T_init=300 K  model_inertia=simscape.enum.onoff.off  planet_inertia=0.001 kg*m^2
      settings: SourceProductBaseCode=LD  LogSimulationData=on
  FWR Ring : fl_lib/Mechanical/Rotational Elements/Inertia  inertia=0.1 kg*m^2  num_ports=foundation.enum.numPorts2.one  w_specify=off  w_priority=High  w=0 rad/s  w_nominal_specify=off  w_nominal_unit=rad/s  w_nominal_value=1  t_specify=off  t_priority=None  t=0 N*m  t_nominal_specify=off  t_nominal_unit=N*m  t_nominal_value=1
  IC : InitialCondition  Value=0
  Ideal Force Sensor : fl_lib/Mechanical/Mechanical Sensors/Ideal Force Sensor
  Ideal Torque Source : fl_lib/Mechanical/Mechanical Sources/Ideal Torque Source
      settings: SourceProductName=Foundation Library
  MRRef : fl_lib/Mechanical/Rotational Elements/Mechanical Rotational Reference
      settings: SourceProductName=Foundation Library
  Mechanical Rotational Reference : fl_lib/Mechanical/Rotational Elements/Mechanical Rotational Reference
  Mechanical Translational Reference : fl_lib/Mechanical/Translational Elements/Mechanical Translational Reference
  PS-Simulink Converter1 : nesl_utility/PS-Simulink Converter  PhysicalDomain=network_engine_domain  SubClassName=ps_output  LeftPortType=input  RightPortType=output  PseudoPeriodic=off  Frequencies=[]  Unit=inherit  AffineConversion=off
  Simulink-PS Converter : nesl_utility/Simulink-PS Converter  PhysicalDomain=network_engine_domain  SubClassName=ps_input  LeftPortType=input  RightPortType=output  PseudoPeriodic=off  Frequencies=[]  NoiseDistribution=none  NoiseParameters=[]  Unit=N  AffineConversion=off  FilteringAndDerivatives=zero  SimscapeFilterOrder=1  InputFilterTimeConstant=0.001  UdotUserProvided=0
  Simulink-PS Converter8 : nesl_utility/Simulink-PS Converter  PhysicalDomain=network_engine_domain  SubClassName=ps_input  LeftPortType=input  RightPortType=output  PseudoPeriodic=off  Frequencies=[]  NoiseDistribution=none  NoiseParameters=[]  Unit=N*m  AffineConversion=off  FilteringAndDerivatives=zero  SimscapeFilterOrder=1  InputFilterTimeConstant=0.001  UdotUserProvided=0
  Solver Configuration4 : nesl_utility/Solver Configuration  PhysicalDomain=network_engine_domain  SubClassName=solver  LeftPortType=input  RightPortType=generic  Tones=[]  Harmonics=[]  SimulateNoise=off  Profile=off  UseLocalSampling=off  EnableSwitchedLinearOptims=on  FrequencyDomain=off  UseCCode=off  RelTol=0.001  AbsTol=1e-06  MinStep=1e-09  ToWorkspace=off  RevertToSquareIcSolve=off  NumHomotopyIterations=100  PhasorMode=off  PhasorModeNumHarmonics=1  DoDC=on  ResidualTolerance=1e-09  UseLocalSolver=off  LocalSolverChoice=NE_BACKWARD_EULER_ADVANCER  LocalSolverSampleTime=0.001  DoFixedCost=off  MaxNonlinIter=3  MaxModeIter=2  ComputeImpulses=off  ImpulseIterations=2  LinearAlgebra=auto  EquationFormulation=NE_TIME_EF  DelaysMemoryBudget=1024  AutomaticFiltering=on  FilteringTimeConstant=0.001  PartitionStorageMethod=AS_NEEDED  PartitionMemoryBudget=1024  PartitionMethod=ROBUST
  BWR Slip : PMIOPort  Side=Right
  BWR : Outport
  wires:
  PS-Simulink Converter1/1 -> BWR/1  "BWR"
  BWR Normal/1 -> Simulink-PS Converter/1
  IC/1 -> Simulink-PS Converter8/1
  FWR Sun/1 -> IC/1
  connections:
  Back Wheel Right/RConn1 -- BWR Slip/RConn1
  Ideal Force Sensor/RConn2 -- PS-Simulink Converter1/LConn1
  Ideal Force Sensor/LConn1 -- Solver Configuration4/RConn1 -- Back Wheel Right/RConn2
  Simulink-PS Converter/RConn1 -- Back Wheel Right/LConn1
  Ideal Force Sensor/RConn1 -- Mechanical Translational Reference/LConn1
  Mechanical Rotational Reference/LConn1 -- FWR Ring/LConn1 -- FWR Planetary Box/RConn1
  MRRef/LConn1 -- Ideal Torque Source/RConn2
  Ideal Torque Source/LConn1 -- FWR Planetary Box/RConn2
  Ideal Torque Source/RConn1 -- Simulink-PS Converter8/RConn1
  FWR Planetary Box/LConn1 -- Back Wheel Right/LConn2

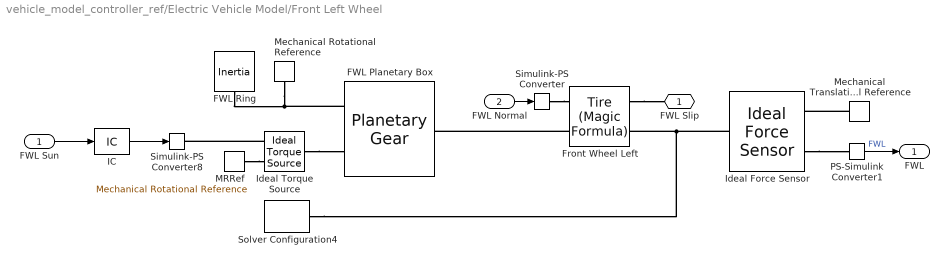
== system vehicle_model_controller_ref/Electric Vehicle Model/Front Left Wheel ==
  FWL Sun : Inport
  FWL Normal : Inport  Port=2
  FWL Planetary Box : sdl_lib/Gears/Planetary Gear  rs_ratio=5.5  friction_model=sdl.enum.gear_friction.none  mu_visc=[0.01, 0.01] N*m/(rad/s)  efficiency=[.96, .98]  temperature_TLU=[280, 300, 320] K  efficiency_sp_TLU=[.95, .9, .85]  efficiency_rp_TLU=[.95, .9, .85]  pwr_thr=[.001, .001] W  thermal_mass=50 J/K  T_init=300 K  model_inertia=simscape.enum.onoff.off  planet_inertia=0.001 kg*m^2
      settings: SourceProductBaseCode=LD  LogSimulationData=on
  FWL Ring : fl_lib/Mechanical/Rotational Elements/Inertia  inertia=0.1 kg*m^2  num_ports=foundation.enum.numPorts2.one  w_specify=off  w_priority=High  w=0 rad/s  w_nominal_specify=off  w_nominal_unit=rad/s  w_nominal_value=1  t_specify=off  t_priority=None  t=0 N*m  t_nominal_specify=off  t_nominal_unit=N*m  t_nominal_value=1
  Front Wheel Left : sdl_lib/Tires & Vehicles/Tire (Magic Formula)  parameterization=sdl.enum.magic_tire_model.peak  F_z1=3000 N  F_x1=3500 N  kappa1=10  B_m=10  C_m=1.9  D_m=1  E_m=0.97  fz0=4000 N  p_Cx=1.685  p_Dx=[1.21, -.037]  p_Ex=[.344, .095, -.02, 0]  p_Kx=[21.51, -.163, .245]  p_Hx=[-.002, .002]  p_Vx=[0, 0]  v_tr_thr=0.1 m/s  r_e=0.3 m  model_compliance=0  stiffness=1e6 N/m  damping=1000 N/(m/s)  model_inertia=0  inertia=1 kg*m^2  initial_velocity=0 rad/s  model_resistance=0  resistance_model=1  coeff=0.015  p_tire=250e3 Pa  alpha=-0.003  beta=0.97  coeff_a=84e-4  coeff_b=6.2e-4 s/m  coeff_c=1.6e-4 s^2/m^2  v_thr=0.001 m/s
  IC : InitialCondition  Value=0
  Ideal Force Sensor : fl_lib/Mechanical/Mechanical Sensors/Ideal Force Sensor
  Ideal Torque Source : fl_lib/Mechanical/Mechanical Sources/Ideal Torque Source
      settings: SourceProductName=Foundation Library
  MRRef : fl_lib/Mechanical/Rotational Elements/Mechanical Rotational Reference
      settings: SourceProductName=Foundation Library
  Mechanical Rotational Reference : fl_lib/Mechanical/Rotational Elements/Mechanical Rotational Reference
  Mechanical Translational Reference : fl_lib/Mechanical/Translational Elements/Mechanical Translational Reference
  PS-Simulink Converter1 : nesl_utility/PS-Simulink Converter  PhysicalDomain=network_engine_domain  SubClassName=ps_output  LeftPortType=input  RightPortType=output  PseudoPeriodic=off  Frequencies=[]  Unit=inherit  AffineConversion=off
  Simulink-PS Converter : nesl_utility/Simulink-PS Converter  PhysicalDomain=network_engine_domain  SubClassName=ps_input  LeftPortType=input  RightPortType=output  PseudoPeriodic=off  Frequencies=[]  NoiseDistribution=none  NoiseParameters=[]  Unit=N  AffineConversion=off  FilteringAndDerivatives=zero  SimscapeFilterOrder=1  InputFilterTimeConstant=0.001  UdotUserProvided=0
  Simulink-PS Converter8 : nesl_utility/Simulink-PS Converter  PhysicalDomain=network_engine_domain  SubClassName=ps_input  LeftPortType=input  RightPortType=output  PseudoPeriodic=off  Frequencies=[]  NoiseDistribution=none  NoiseParameters=[]  Unit=N*m  AffineConversion=off  FilteringAndDerivatives=zero  SimscapeFilterOrder=1  InputFilterTimeConstant=0.001  UdotUserProvided=0
  Solver Configuration4 : nesl_utility/Solver Configuration  PhysicalDomain=network_engine_domain  SubClassName=solver  LeftPortType=input  RightPortType=generic  Tones=[]  Harmonics=[]  SimulateNoise=off  Profile=off  UseLocalSampling=off  EnableSwitchedLinearOptims=on  FrequencyDomain=off  UseCCode=off  RelTol=0.001  AbsTol=1e-06  MinStep=1e-09  ToWorkspace=off  RevertToSquareIcSolve=off  NumHomotopyIterations=100  PhasorMode=off  PhasorModeNumHarmonics=1  DoDC=on  ResidualTolerance=1e-09  UseLocalSolver=off  LocalSolverChoice=NE_BACKWARD_EULER_ADVANCER  LocalSolverSampleTime=0.001  DoFixedCost=off  MaxNonlinIter=3  MaxModeIter=2  ComputeImpulses=off  ImpulseIterations=2  LinearAlgebra=auto  EquationFormulation=NE_TIME_EF  DelaysMemoryBudget=1024  AutomaticFiltering=on  FilteringTimeConstant=0.001  PartitionStorageMethod=AS_NEEDED  PartitionMemoryBudget=1024  PartitionMethod=ROBUST
  FWL Slip : PMIOPort  Side=Left
  FWL : Outport
  wires:
  PS-Simulink Converter1/1 -> FWL/1  "FWL"
  FWL Normal/1 -> Simulink-PS Converter/1
  IC/1 -> Simulink-PS Converter8/1
  FWL Sun/1 -> IC/1
  connections:
  Front Wheel Left/RConn1 -- FWL Slip/RConn1
  Front Wheel Left/LConn2 -- FWL Planetary Box/LConn1
  Ideal Torque Source/LConn1 -- FWL Planetary Box/RConn2
  Ideal Force Sensor/RConn2 -- PS-Simulink Converter1/LConn1
  Ideal Force Sensor/LConn1 -- Solver Configuration4/RConn1 -- Front Wheel Left/RConn2
  Simulink-PS Converter/RConn1 -- Front Wheel Left/LConn1
  Mechanical Translational Reference/LConn1 -- Ideal Force Sensor/RConn1
  MRRef/LConn1 -- Ideal Torque Source/RConn2
  Ideal Torque Source/RConn1 -- Simulink-PS Converter8/RConn1
  Mechanical Rotational Reference/LConn1 -- FWL Ring/LConn1 -- FWL Planetary Box/RConn1
